simulink model "prioritydemo_org"  (Simulink 10.0)
settings: Solver=VariableStepDiscrete  StartTime=0.0  StopTime=inf  RelTol=1e-3  EnableMultiTasking=on
undefined symbols (not defined in the file): gcbh
Description:
  | Block Priority
  | 
  | This model shows what happens when blocks are assigned different
  | priorities.  The block priority affects the order in which the blocks are
  | executed.  You can set the block priority through the Block Properties dialog.
  | 
  | The block sorting order is calculated only at the beginning of a
  | simulation.  For this reason, changes to a block's Priority property are only
  | updated when the simulation is started.  Double click on the green block
  | to change the priority levels for the blocks and see what happens.
  | 
  | Inside of each triggered subsystem is an S-Function which controls the coloring
  | of the blocks and also slows down the simulation. The priority level of the block
  | is displayed using the format attribute string that can be set in the Block Properties
  | dialog.
settings Model: Creator=The MathWorks, Inc.  LastModifiedBy=bhisma  ExtModeTrigMode=oneshot  ExtModeArmWhenConnect=off  ExtModeAutoUpdateStatusClock=off
settings DataIOCC: ReturnWorkspaceOutputs=on
settings OptimizationCC: BlockReduction=off  BooleanDataType=off  ExpressionDepthLimit=2147483647  InitFltsAndDblsToZero=on  BufferReusableBoundary=off
settings DebuggingCC: SaveWithParameterizedLinksMsg=none  UnderspecifiedInitializationDetection=Simplified  MergeDetectMultiDrivingBlocksExec=error  SignalResolutionControl=TryResolveAllWithWarning  MultiTaskDSMMsg=warning  MultiTaskCondExecSysMsg=none  IntegerOverflowMsg=none  FcnCallInpInsideContextMsg=warning  BusObjectLabelMismatch=none  AllowSymbolicDim=off  StateNameClashWarn=warning  IntegerSaturationMsg=none
settings HardwareCC: TargetUnknown=on
settings GRTTargetCC: TargetFcnLib=ansi_tfl_tmw.mat  GeneratePreprocessorConditionals=Disable all
settings ConfigComp: CovExternalEMLEnable=off

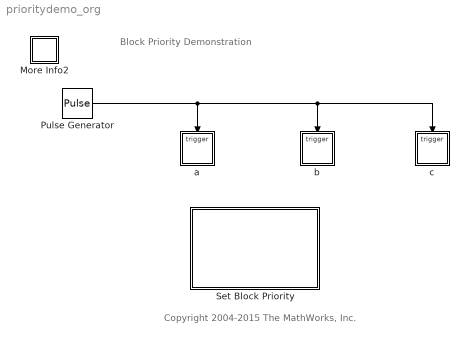
== system prioritydemo_org ==
  note: Block Priority Demonstration
  note: Copyright 2004-2015 The MathWorks, Inc.
  More Info2 : Subsystem
      settings: OpenFcn=showdemo(bdroot(gcs))
      mask Display: disp('?')
  Pulse Generator : DiscretePulseGenerator
  Set Block Priority : Subsystem  StartFcn=set_param(gcbh,'MaskEnables',{'off'})  StopFcn=set_param(gcbh,'MaskEnables',{'on'})  mask(Set Block Priority){PriorityOrder=1 2 3}
      mask prompts: PriorityOrder "Priority order:"
      mask help: This block lets you select the priority that is used on the three triggered subsystems above it. The priority may only be set when the simulation is stopped.
      mask init:
      | spriorityfcn([],[],[],'PriorityOrder');
      mask TypeOptions PriorityOrder: 1 2 3 | 1 3 2 | 2 1 3 | 2 3 1 | 3 1 2 | 3 2 1
      mask Display: disp(['Set\nBlock\nPriority\n' PriorityOrder])
  a : Subsystem  Priority=1
      settings: AttributesFormatString=Priority: %<Priority>
  b : Subsystem  Priority=2
      settings: AttributesFormatString=Priority: %<Priority>
  c : Subsystem  Priority=3
      settings: AttributesFormatString=Priority: %<Priority>
  wires:
  Pulse Generator/1 -> c/Trigger, b/Trigger, a/Trigger

== system prioritydemo_org/More Info2 ==

== system prioritydemo_org/Set Block Priority ==

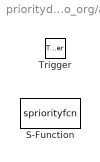
== system prioritydemo_org/a ==
  Trigger : TriggerPort  VariantControl=(inherit)
  S-Function : S-Function  FunctionName=spriorityfcn  SFunctionDeploymentMode=off  EnableBusSupport=off

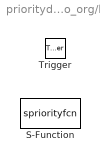
== system prioritydemo_org/b ==
  Trigger : TriggerPort  VariantControl=(inherit)
  S-Function : S-Function  FunctionName=spriorityfcn  SFunctionDeploymentMode=off  EnableBusSupport=off

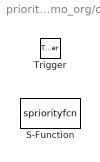
== system prioritydemo_org/c ==
  Trigger : TriggerPort  VariantControl=(inherit)
  S-Function : S-Function  FunctionName=spriorityfcn  SFunctionDeploymentMode=off  EnableBusSupport=off
